simulink library "csc_kfl_kalman_filter_lib"  (R2015b)
settings: Solver=ode45  SolverMode=SingleTasking  StartTime=0.0  StopTime=10.0  RelTol=1e-3
libraries: util_info_lib x2, csc_ekf_nonlinear_filter_lib x2, csc_snp_sensor_prep_lib x2
settings Model: ExtModeAutoUpdateStatusClock=off  Creator=Administrator  LastModifiedBy=Mark Agbayani
settings DataIOCC: SaveFormat=Array  SignalLoggingSaveFormat=ModelDataLogs
settings OptimizationCC: BlockReduction=off  BooleanDataType=off  ExpressionDepthLimit=2147483647
settings DebuggingCC: SaveWithParameterizedLinksMsg=none  UnderspecifiedInitializationDetection=Classic  MergeDetectMultiDrivingBlocksExec=none  SignalResolutionControl=TryResolveAllWithWarning  FcnCallInpInsideContextMsg=EnableAllAsWarning  StateNameClashWarn=warning  StrictBusMsg=Warning
settings HardwareCC: ProdBitPerPointer=32  ProdLargestAtomicFloat=None  ProdIntDivRoundTo=Undefined  ProdEndianess=Unspecified  ProdWordSize=32  ProdHWDeviceType=32-bit Generic  TargetUnknown=on
settings GRTTargetCC: GeneratePreprocessorConditionals=Disable all  CombineOutputUpdateFcns=off  GRTInterface=on
settings ConfigComp: CovModelRefEnable=Off  CovSFcnEnable=off

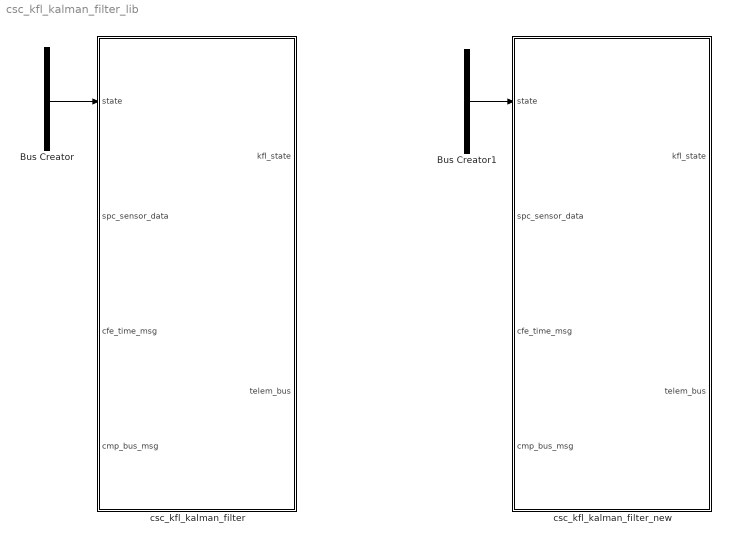
== system csc_kfl_kalman_filter_lib ==
  Bus Creator : BusCreator  Inputs=4
  Bus Creator1 : BusCreator  Inputs=5
  csc_kfl_kalman_filter : Subsystem
  csc_kfl_kalman_filter_new : Subsystem
  wires:
  Bus Creator/1 -> csc_kfl_kalman_filter/1(state)
  ? -> Bus Creator/1  "x"
  ? -> Bus Creator/2  "accel"
  ? -> Bus Creator/3  "rate"
  ? -> Bus Creator/4  "q"
  Bus Creator1/1 -> csc_kfl_kalman_filter_new/1(state)
  ? -> Bus Creator1/1  "x"
  ? -> Bus Creator1/2  "accel"
  ? -> Bus Creator1/3  "rate"
  ? -> Bus Creator1/4  "q"
  ? -> Bus Creator1/5  "altitude"

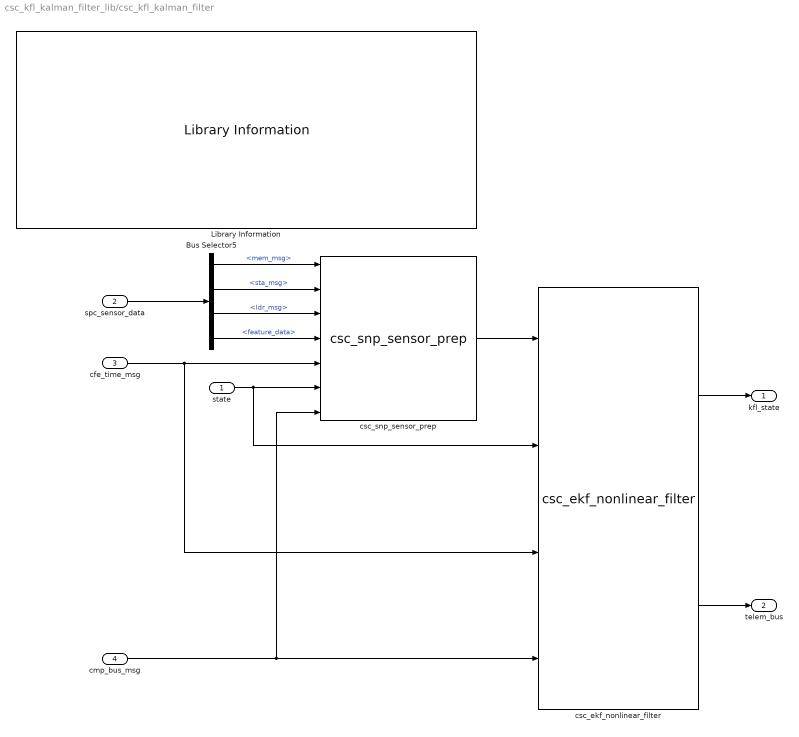
== system csc_kfl_kalman_filter_lib/csc_kfl_kalman_filter ==
  state : Inport
  spc_sensor_data : Inport  Port=2
  cfe_time_msg : Inport  Port=3
  cmp_bus_msg : Inport  Port=4
  Bus Selector5 : BusSelector  OutputSignals=mem_msg,sta_msg,ldr_msg,feature_data
  Library Information : util_info_lib/Library Information  owner='NONE'
  csc_ekf_nonlinear_filter : csc_ekf_nonlinear_filter_lib/csc_ekf_nonlinear_filter
  csc_snp_sensor_prep : csc_snp_sensor_prep_lib/csc_snp_sensor_prep
  kfl_state : Outport
  telem_bus : Outport  Port=2
  wires:
  Bus Selector5/2 -> csc_snp_sensor_prep/2  "<sta_msg>"
  csc_ekf_nonlinear_filter/2 -> telem_bus/1
  Bus Selector5/1 -> csc_snp_sensor_prep/1  "<mem_msg>"
  Bus Selector5/4 -> csc_snp_sensor_prep/4  "<feature_data>"
  Bus Selector5/3 -> csc_snp_sensor_prep/3  "<ldr_msg>"
  spc_sensor_data/1 -> Bus Selector5/1
  csc_snp_sensor_prep/1 -> csc_ekf_nonlinear_filter/1
  cfe_time_msg/1 -> csc_snp_sensor_prep/5, csc_ekf_nonlinear_filter/3
  state/1 -> csc_ekf_nonlinear_filter/2, csc_snp_sensor_prep/6
  csc_ekf_nonlinear_filter/1 -> kfl_state/1
  cmp_bus_msg/1 -> csc_snp_sensor_prep/7, csc_ekf_nonlinear_filter/4

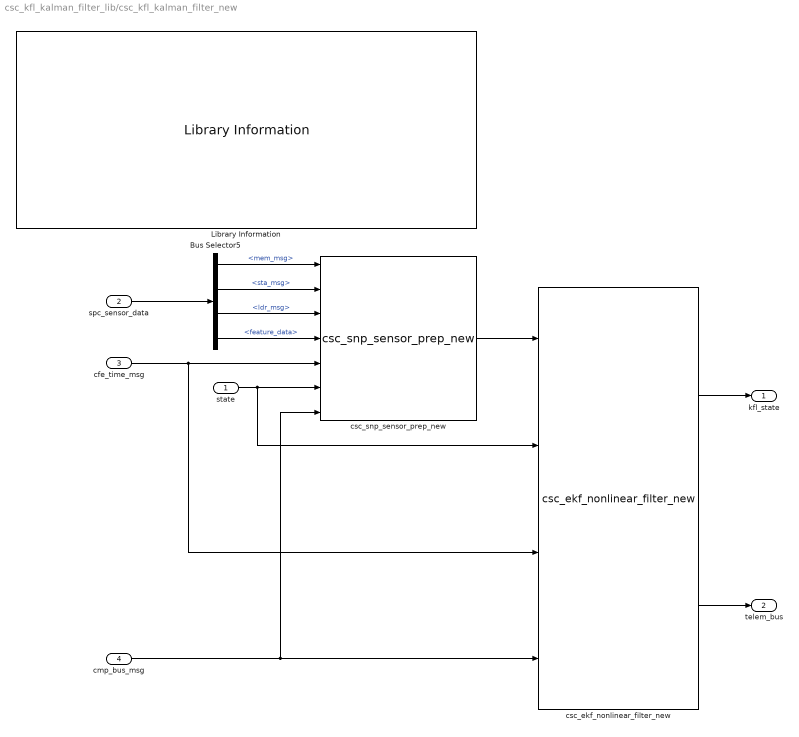
== system csc_kfl_kalman_filter_lib/csc_kfl_kalman_filter_new ==
  state : Inport
  spc_sensor_data : Inport  Port=2
  cfe_time_msg : Inport  Port=3
  cmp_bus_msg : Inport  Port=4
  Bus Selector5 : BusSelector  OutputSignals=mem_msg,sta_msg,ldr_msg,feature_data
  Library Information : util_info_lib/Library Information  owner='NONE'
  csc_ekf_nonlinear_filter_new : csc_ekf_nonlinear_filter_lib/csc_ekf_nonlinear_filter_new
  csc_snp_sensor_prep_new : csc_snp_sensor_prep_lib/csc_snp_sensor_prep_new
  kfl_state : Outport
  telem_bus : Outport  Port=2
  wires:
  Bus Selector5/2 -> csc_snp_sensor_prep_new/2  "<sta_msg>"
  csc_ekf_nonlinear_filter_new/2 -> telem_bus/1
  Bus Selector5/1 -> csc_snp_sensor_prep_new/1  "<mem_msg>"
  Bus Selector5/4 -> csc_snp_sensor_prep_new/4  "<feature_data>"
  Bus Selector5/3 -> csc_snp_sensor_prep_new/3  "<ldr_msg>"
  spc_sensor_data/1 -> Bus Selector5/1
  csc_snp_sensor_prep_new/1 -> csc_ekf_nonlinear_filter_new/1
  cfe_time_msg/1 -> csc_ekf_nonlinear_filter_new/3, csc_snp_sensor_prep_new/5
  state/1 -> csc_ekf_nonlinear_filter_new/2, csc_snp_sensor_prep_new/6
  csc_ekf_nonlinear_filter_new/1 -> kfl_state/1
  cmp_bus_msg/1 -> csc_snp_sensor_prep_new/7, csc_ekf_nonlinear_filter_new/4
